simulink model "blockdemo"  (Simulink 6.3)
settings: Solver=FixedStepDiscrete  StartTime=0  StopTime=100  FixedStep=1  RelTol=1e-3
InitFcn:
  | %% DSPBuilder Start
  | alt_dspbuilder_update_model(bdroot)
  | %% DSPBuilder End
libraries: allblocks_alteradspbuilder2 x8, simulink x1
settings Model: Creator=mjervis  LastModifiedBy=delphick
settings OptimizationCC: BooleanDataType=off  InlineInvariantSignals=on
settings DebuggingCC: SolverPrmCheckMsg=none
settings HardwareCC: TargetUnknown=on

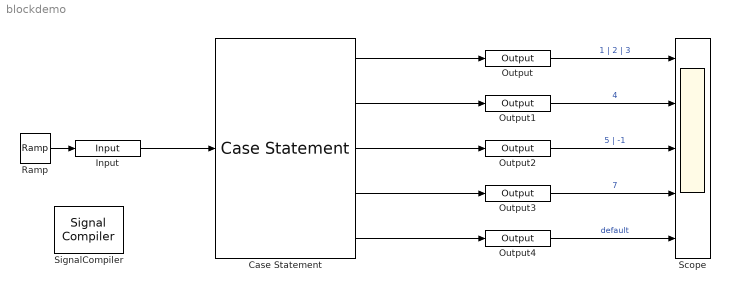
== system blockdemo ==
  Case Statement : allblocks_alteradspbuilder2/Case Statement  numOutputs=5  case_expression=1|2|3,4,5|-1,7  formatted_case_expression=00000001 00000010 00000011,00000100,00000101 11111111,00000111  BusType=Signed Integer  bwl=8  bwr=0  pipeline=off  hasDefault=on
  Input : allblocks_alteradspbuilder2/Input  iofile=C:\workspace_clean\Documentation\DesignExamples\Tutorials\UnitBlocks\GateAndControl\CaseStatement\tb_blockdemo\blockdemo_Input.salt  BusType=Signed Integer  bwl=6  bwr=0  SpecifyClock=off  PORTTYPE=Input
  Output : allblocks_alteradspbuilder2/Output  iofile=C:\workspace_clean\Documentation\DesignExamples\Tutorials\UnitBlocks\GateAndControl\CaseStatement\tb_blockdemo\blockdemo_Output.capture  BusType=Single Bit  bwl=8  bwr=0  PORTTYPE=Output
  Output1 : allblocks_alteradspbuilder2/Output  iofile=C:\workspace_clean\Documentation\DesignExamples\Tutorials\UnitBlocks\GateAndControl\CaseStatement\tb_blockdemo\blockdemo_Output1.capture  BusType=Single Bit  bwl=8  bwr=0  PORTTYPE=Output
  Output2 : allblocks_alteradspbuilder2/Output  iofile=C:\workspace_clean\Documentation\DesignExamples\Tutorials\UnitBlocks\GateAndControl\CaseStatement\tb_blockdemo\blockdemo_Output2.capture  BusType=Single Bit  bwl=8  bwr=0  PORTTYPE=Output
  Output3 : allblocks_alteradspbuilder2/Output  iofile=C:\workspace_clean\Documentation\DesignExamples\Tutorials\UnitBlocks\GateAndControl\CaseStatement\tb_blockdemo\blockdemo_Output3.capture  BusType=Single Bit  bwl=8  bwr=0  PORTTYPE=Output
  Output4 : allblocks_alteradspbuilder2/Output  iofile=C:\workspace_clean\Documentation\DesignExamples\Tutorials\UnitBlocks\GateAndControl\CaseStatement\tb_blockdemo\blockdemo_Output4.capture  BusType=Single Bit  bwl=8  bwr=0  PORTTYPE=Output
  Ramp : simulink/Sources/Ramp  slope=1  start=0  X0=0
  Scope : Scope  NumInputPorts=5
      settings: YMin=-0.5~-0.5~-0.5~-0.5~-0.5  YMax=1.5~1.5~1.5~1.5~1.5  SampleInput=on
  SignalCompiler : allblocks_alteradspbuilder2/Signal Compiler  DeviceFamily=Stratix IV  DeviceName=AUTO  EnableSignalTap=off  SignalTapDepth=128  UseBoardBlock=off  StpUseDefaultClock=on  StpClock=clock
  wires:
  Ramp/1 -> Input/1
  Input/1 -> Case Statement/1
  Case Statement/1 -> Output/1
  Case Statement/2 -> Output1/1
  Case Statement/3 -> Output2/1
  Case Statement/4 -> Output3/1
  Case Statement/5 -> Output4/1
  Output/1 -> Scope/1  "1 | 2 | 3"
  Output1/1 -> Scope/2  "4"
  Output2/1 -> Scope/3  "5 | -1"
  Output3/1 -> Scope/4  "7"
  Output4/1 -> Scope/5  "default"
